simulink model "Week1_pr7"  (R2020b)
settings: Solver=VariableStepAuto  StartTime=0.0  StopTime=10.0  RelTol=1e-3
settings Model: Creator=user  LastModifiedBy=user

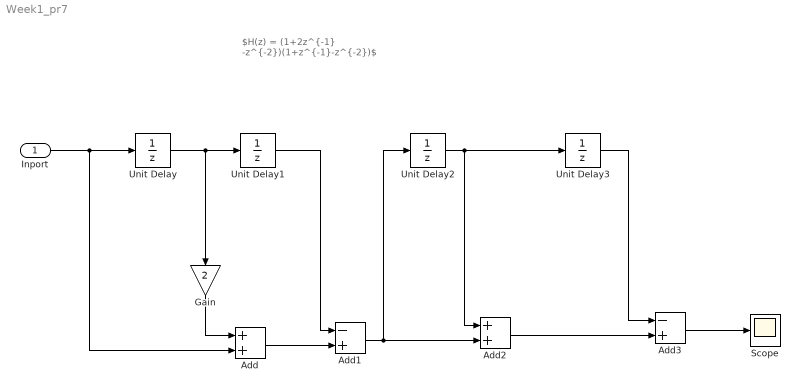
== system Week1_pr7 ==
  note: $H(z) = (1+2z^{-1} -z^{-2})(1+z^{-1}-z^{-2})$
  Inport : Inport
  Add : Sum
  Add1 : Sum  Inputs=-+
  Add2 : Sum
  Add3 : Sum  Inputs=-+
  Gain : Gain  Gain=2
  Scope : Scope
  Unit Delay{,1..3} (4 alike) : UnitDelay  SampleTime=-1  HasFrameUpgradeWarning=on
  wires:
  Add3/1 -> Scope/1
  Inport/1 -> Add/2, Unit Delay/1
  Gain/1 -> Add/1
  Add1/1 -> Add2/2, Unit Delay2/1
  Unit Delay2/1 -> Add2/1, Unit Delay3/1
  Unit Delay3/1 -> Add3/1
  Unit Delay/1 -> Gain/1, Unit Delay1/1
  Unit Delay1/1 -> Add1/1
  Add2/1 -> Add3/2
  Add/1 -> Add1/2
